simulink library "LinWindVel2D_ul"  (R2020a)
settings: Solver=VariableStepAuto  StartTime=0.0  StopTime=10.0  RelTol=1e-3
undefined symbols (not defined in the file): Env
settings Model: Creator=John Jr  LastModifiedBy=John Jr
settings SFSimCC: CustomCodeUndefinedFunction=UseInterfaceOnly

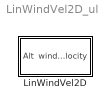
== system LinWindVel2D_ul ==
  LinWindVel2D : Subsystem  mask{v0=Env.wind0.Value, m=Env.windSlope.Value}
      mask prompts: v0 "Wind speed at ground level [m/s]"; m "Wind speed slope [m/s/m]"
      mask DialogControl DescTextVar Prompt: This subsystem calculates the wind speed at the current input altitude. The wind speed is modeled as a linear function of altitude.
      mask Display:
      | patch([0 1 1 0], [0 0 1 1],[.8 1 1])
      | 
      | port_label('input',1,'z [m]','texmode','on')
      | 
      | port_label('output',1,'v_w [m/s]','texmode','on')

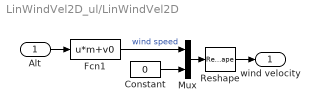
== system LinWindVel2D_ul/LinWindVel2D ==
  Alt : Inport
  Constant : Constant  Value=0
  Fcn1 : Fcn  Expr=u*m+v0
  Mux : Mux  Inputs=2
  Reshape : Reshape  OutputDimensionality=Column vector (2-D)
  wind velocity : Outport  VectorParamsAs1DForOutWhenUnconnected=off
  wires:
  Alt/1 -> Fcn1/1
  Fcn1/1 -> Mux/1  "wind speed"
  Constant/1 -> Mux/2
  Mux/1 -> Reshape/1
  Reshape/1 -> wind velocity/1
